simulink model "sim_all_2019b"  (R2019b)
settings: Solver=VariableStepAuto  StartTime=0.0  StopTime=2000  RelTol=1e-3
values from neighbouring files (symbols this model uses):
  nav_DT = 0.1    [navigation.m]
  nav_giro = 2    [navigation.m]
  nav_h0 = 0    [navigation.m]
  nav_lat0 = cornerC(1)    [navigation.m]
  nav_lon0 = cornerC(2)    [navigation.m]
  nav_plane_AB = coefficient_plane(nav_A,nav_B)    [navigation.m]
  nav_plane_BC = coefficient_plane(nav_B,nav_C)    [navigation.m]
  nav_plane_CD = coefficient_plane(nav_C,nav_D)    [navigation.m]
  nav_plane_DA = coefficient_plane(nav_D,nav_A)    [navigation.m]
undefined symbols (not defined in the file or in its folder): a1, a2, alpha1, alpha2, cornerA, cornerB, cornerC, cornerD, ctrl_clockwise, ctrl_int_bound_or, ctrl_int_bound_pos, ctrl_k_or, ctrl_k_pos, ctrl_Ki_vel, ctrl_Kp_v_pos, ctrl_Kp_vel, ctrl_TAM, ctrl_Ts, ctrl_va_uncontrolled, ctrl_vel_uncontrolled, D, dead_zone_limit, depth, DiscIntNeverNeededParam, distanceFromWall, initInspectedSide, initPoint, mod_A, mod_Cd_F, mod_Cd_M, mod_eta_init, mod_g, mod_h0, mod_Ixx, mod_Iyy, mod_Izz, mod_Kp_dot, mod_lat0, mod_lon0, mod_m, mod_Mq_dot, mod_ni_init, mod_Nr_dot, mod_p1, mod_p2, mod_p3, mod_p4, mod_p5, mod_p6, mod_R, mod_Rm, mod_t1, mod_t2, mod_t3, mod_t4, mod_t5, mod_t6, mod_W, mod_Xu_dot, mod_Yv_dot ... (+44)
libraries: simulink x8, cstblocks x6, simulink_extras x1
(part 4 of 6)

== matlab function sim_all_2019b/Mission_supervisor_v3/Mission_Supervisor/Completamento/MATLAB Function ==
  data: delta_current_comp output; parete input; delta_stato_comp output; Pos_d output size=3; Vel_d output; Dpp_d output; Orp_d output; Pos_s input; Vel_s input; Dpp_s input; Dps_s input; Orp_s input; depth parameter; speed parameter; distanceFromWall parameter; relativeDirection parameter; dps_fin input; error_flag input; soglia_SOS_vel parameter; soglia_parete_frenata parameter; soglia_SOS_orp parameter; soglia_SOS_pos parameter; soglia_SOS_parete parameter; SOS parameter; giro input
function [delta_current_comp, delta_stato_comp, Pos_d, Vel_d, Dpp_d, Orp_d] = Completamento(parete, Pos_s, Vel_s, Dpp_s, Dps_s, Orp_s, depth, speed, distanceFromWall, relativeDirection, dps_fin, error_flag, soglia_SOS_vel, soglia_parete_frenata, soglia_SOS_orp, soglia_SOS_pos, soglia_SOS_parete, SOS, giro)

    disp("Completamento del pattugliamento parziale della parete " + parete);
    
    %% Unità di misura 
    
    % Pos_d, Pos_s, soglia_SOS_pos                                                                              [deg, deg, m]
    % Orp_d, Orp_s, soglia_SOS_orp                                                                              [rad]
    % relativeDirection                                                                                         [deg]
    % Dpp_d, Dps_d, Dpp_s, Dps_s, dps_fin, distanceFromWall, depth, soglia_SOS_parete, soglia_parete_frenata    [m]
    % Vel_d, Vel_s, speed, soglia_SOS_vel                                                                       [m/s]

    %% Inizializzazione variabili
    
    % Utilizzata per permanere in questo stato e inizializzata a zero
    % perché fuori dal ciclo
    delta_stato_comp = 0; 
    
    pronti = false;
    
    
    %% Preparazione dei riferimenti da fornire ai blocchi successivi
    
    % Profondità da mantenere
    Pos_d = [nan; nan; depth];
                                                                            %*****TEST******%
                                                                            %Pos_d = [nan; nan; 0];
    
    % Velocità da raggiungere
    Vel_d = speed;              
                                                                            %*****TEST******%
                                                                            %Vel_d_vett = [0; 0; 0];

    % Distanza dalla parete da mantenere
    Dpp_d = distanceFromWall;
    
    % Orientazione da mantenere
    Orp_d = deg2rad(relativeDirection);
        
    % Transizione di stato effettiva
    delta_current_comp = 204 - 203;  
  
    %% Verifiche
    
    % Verifica sulla corretta profondità, orientazione, distanza dalla parete pattugliata 
    % e velocità
    if (abs(Pos_s(3) - Pos_d(3)) > soglia_SOS_pos(3) || ...
        abs(Orp_s - Orp_d) > soglia_SOS_orp || ...
        abs(Dpp_s - Dpp_d) > soglia_SOS_parete || ...
        norm(Vel_s) - Vel_d > soglia_SOS_vel)
    
        SOS = 1;
        disp("EMERGENZA:");
        
        if (abs(Orp_s - Orp_d) > soglia_SOS_orp)
            disp("Rilevato errore sull'orientazione relativa");
        end
        
        if (abs(Dpp_s - Dpp_d) > soglia_SOS_parete)
            disp("Rilevato errore sulla distanza da parete");
        end
        
        if (abs(Pos_s(3) - Pos_d(3)) > soglia_SOS_pos(3))
            disp("Rilevato errore sulla profondita Z");
        end
        
        if (norm(Vel_s) - Vel_d > soglia_SOS_vel)
            disp("Rilevato errore nella velocita");
        end

    end
    
                                                                            %*****TEST******%
                                                                            % if(contatore > 1)
                                                                            %     error_flag = 1;
                                                                            % end

     if error_flag == 1
        disp("EMERGENZA: errore segnalato dagli altri sottosistemi");
        SOS = 1;
     end
     
                                                                            %*****TEST******%
                                                                            %dps_fin = 4;

    % Si verifica di pattugliare alla velocità desiderata fino al punto di
    % frenata
    if (SOS == 0 && ...
        abs(Dps_s - (dps_fin + 3*speed)) < soglia_parete_frenata) % Analogo a quanto detto in "Pattugliamento"
    
        pronti = true;
        
    end
    
    %% Decisione dello stato successivo
    
    if pronti == true
        
        delta_stato_comp = 205 - 204; % Transizione eseguita correttamente
    end
    if SOS == 1
            
            delta_stato_comp = 301 - 204; % Transizione nello stato di emergenza
    end
  % Si rimane nello stato corrente.

end

== matlab function sim_all_2019b/Mission_supervisor_v3/Mission_Supervisor/Frenata in completamento/MATLAB Function ==
  data: delta_current_fren_comp output; delta_stato_fren_comp output; SOS_205 output; Pos_d output size=3; Dpp_d output; Dps_d output; Orp_d output; Pos_s input; Orp_s input; Dpp_s input; Dps_s input; depth parameter; distanceFromWall parameter; relativeDirection parameter; dps_fin input; error_flag input; soglia_SOS_pos parameter; soglia_SOS_parete parameter; soglia_SOS_orp parameter; soglia_parete parameter; SOS parameter
function [delta_current_fren_comp, delta_stato_fren_comp, SOS_205, Pos_d, Dpp_d, Dps_d, Orp_d] = Frenata_completamento(Pos_s, Orp_s, Dpp_s, Dps_s, depth, distanceFromWall, relativeDirection, dps_fin, error_flag, soglia_SOS_pos, soglia_SOS_parete, soglia_SOS_orp, soglia_parete, SOS)

    disp("Frenata (durante il completamento del pattugliamento parziale)");
    
    %% Unità di misura 
    
    % Pos_d, Pos_s, soglia_SOS_pos                                                                      [deg, deg, m]
    % Orp_d, Orp_s, soglia_SOS_orp                                                                      [rad]
    % relativeDirection                                                                                 [deg]
    % Dpp_d, Dps_d, Dpp_s, Dps_s, dps_fin, distanceFromWall, depth, soglia_SOS_parete, soglia_parete    [m]
    
    %% Inizializzazione variabili
    
    delta_stato_fren_comp = 0;
    
    pronti = false;
    

    %% Preparazione dei riferimenti da fornire si blocchi successivi
    
    % Profondità da mantenere
    Pos_d = [nan; nan; depth];
                                                                            %*****TEST******%
                                                                            %Pos_d = [nan;nan;0];
    % Distanza dalla parete da mantenere
    Dpp_d = distanceFromWall;
    Dps_d = dps_fin;
    
    % Orientazione da mantenere
    Orp_d = deg2rad(relativeDirection);
    
    % Transizione di stato effettiva
    delta_current_fren_comp = 205 - 204;  
    
       
    %% Verifiche

    % Si verifica la corretta orientazione, profondità e distanza dalla parete di pattugliamento 
    if (abs(Pos_s(3) - Pos_d(3)) > soglia_SOS_pos(3) || ...
        abs(Orp_s - Orp_d) > soglia_SOS_orp || ...
        abs(Dpp_s - Dpp_d) > soglia_SOS_parete)
    
        SOS = 1;
        pronti = true;
        disp("EMERGENZA:");
        
        if (abs(Pos_s(3) - Pos_d(3)) > soglia_SOS_pos(3))
            disp("Rilevato errore sulla profondita Z");
        end
        
        if (abs(Orp_s - Orp_d) > soglia_SOS_orp)
            disp("Rilevato errore sull'orientazione relativa");
        end
        
        if (abs(Dpp_s - Dpp_d) > soglia_SOS_parete)
            disp("Rilevato errore sulla distanza da parete");
        end
    end
    
    if error_flag == 1
        disp("EMERGENZA: errore segnalato dagli altri sottosistemi");
        SOS = 1;
    end
 
    SOS_205 = SOS;                                                                     %*****TEST******%
                                                                            %dps_fin = 8;

    % Si verifica di aver raggiunto la posizione desiderata di fine pattugliamento
    if (SOS==0 && ...
        abs(Dps_s - dps_fin) < soglia_parete) 
        pronti = true;
        
    end
    
    %% Decisione dello stato successivo
    
    if (pronti == true || SOS == 1)
        
        delta_stato_fren_comp = 301 - 205; % Transizione di stato
    end
    % Si rimane nello stato corrente
    

end

== matlab function sim_all_2019b/Mission_supervisor_v3/Mission_Supervisor/Orientazione in superficie/MATLAB Function ==
  data: delta_current_or_sup output; delta_stato_or_sup output; Or_in input; error_flag input; punto_iniz_patt input; SOS parameter; Pos_d output size=3; Or_d output size=3; soglia_SOS_pos parameter; soglia_or parameter; Pos_s input; Or_s input; soglia_SOS_or parameter
function [delta_current_or_sup, delta_stato_or_sup, Pos_d, Or_d] = Orientazioneinsuperficie(Or_in, error_flag, punto_iniz_patt, SOS, soglia_SOS_pos, soglia_or, Pos_s, Or_s, soglia_SOS_or)

    disp("Orientazione in superficie");
    
    %% Unità di misura 
    
    % Pos_d, Pos_s, soglia_SOS_pos, punto_iniz_patt                             [deg,deg,m]
    % Or_d, Or_in, Or_s, soglia_SOS_or, soglia_or                               [deg,deg,deg]

    %% Inizializzazione variabili
    
    delta_stato_or_sup = 0;
    
    pronti = false; 

    %% Preparazione dei riferimenti da fornire ai blocchi successivi
  
    % Posizione da mantenere
    Pos_d = punto_iniz_patt; 
                                                                            %*****TEST******%
                                                                            %Pos_d = [43; 11; 0];  
    % Orientazione desiderata e necessaria per raggiungere
    % il punto di rientro
    Or_d = Or_in;
                                                                            %*****TEST******%
                                                                            %Or_d = [1; 1; 1];
  
    % Transizione di stato effettiva
    delta_current_or_sup = 302 - 301;
   
    
    %% Verifiche 
    
    % Verifica della posizione e dell'orientazione
   if (abs(Pos_s(1) - Pos_d(1)) > soglia_SOS_pos(1) || ...
       abs(Pos_s(2) - Pos_d(2)) > soglia_SOS_pos(2) || ...
       abs(Pos_s(3) - Pos_d(3)) > soglia_SOS_pos(3) || ...
       abs(Or_s(1) - Or_d(1)) > soglia_SOS_or(1) || ...
       abs(Or_s(2) - Or_d(2)) > soglia_SOS_or(2))
    
        SOS = 1;
        disp("EMERGENZA:");
        
        
        if (abs(Pos_s(1) - Pos_d(1)) > soglia_SOS_pos(1))
            disp("Rilevato errore sulla posizione X");
        end
        if (abs(Pos_s(2) - Pos_d(2)) > soglia_SOS_pos(2))
            disp("Rilevato errore sulla posizione Y");
        end
        if (abs(Pos_s(3) - Pos_d(3)) > soglia_SOS_pos(3))
            disp("Rilevato errore sulla profondita Z");
        end
        if (abs(Or_s(1) - Or_d(1)) > soglia_SOS_or(1))
            disp("Rilevato errore sulla rotazione di roll");
        end
        if (abs(Or_s(2) - Or_d(2)) > soglia_SOS_or(2))
            disp("Rilevato errore sulla rotazione di pitch");
        end

    end
    
    if error_flag == 1
        disp("EMERGENZA: errore segnalato dagli altri sottosistemi");
        SOS = 1;
    end
    
    % Si verifica di aver raggiunto l'orientazione desiderata
    if  (SOS == 0 && ...
         abs(Or_s(3) - Or_d(3)) < soglia_or(3))
    
        pronti = true;
        
    end
    
%% Decisione dello stato successivo
    
    if pronti == true
       
        delta_stato_or_sup = 303 - 302; % Transizione eseguita correttamente
    end
    
    if SOS == 1
            
            delta_stato_or_sup = 304 - 302; % Transizione nello stato di emergenza
    end

    % Si rimane nello stato corrente
end

== matlab function sim_all_2019b/Mission_supervisor_v3/Mission_Supervisor/Pattugliamento/MATLAB Function ==
  data: parete input; contatore input; delta_current_patt output; Pos_s input; Dpp_s input; Dps_s input; delta_stato_patt output; Pos_d output size=3; Vel_d output; Dpp_d output; Orp_d output; Orp_s input; Vel_s input; depth parameter; speed parameter; distanceFromWall parameter; relativeDirection parameter; soglia_parete_frenata parameter; soglia_SOS_orp parameter; soglia_SOS_parete parameter; soglia_SOS_pos parameter; error_flag input; SOS parameter; soglia_SOS_vel parameter; giro input
function [delta_current_patt, delta_stato_patt, Pos_d, Vel_d, Dpp_d, Orp_d] = Pattugliamento(parete, contatore, Pos_s, Dpp_s, Dps_s, Orp_s, Vel_s, depth, speed, distanceFromWall, relativeDirection, soglia_parete_frenata, soglia_SOS_orp, soglia_SOS_parete, soglia_SOS_pos, error_flag, SOS, soglia_SOS_vel, giro)
    
    % In base al valore del contatore un display mostra il tipo di pattugliamento (parziale o completo)
    if contatore == 0
        disp("Pattugliamento parziale parete " + parete);
    else
        disp("Pattugliamento parete " + parete);
    end 
    
    %% Unità di misura 
    
    % Pos_d, Pos_s, soglia_SOS_pos                                                        [deg, deg, m]
    % Orp_d, Orp_s, soglia_SOS_orp                                                        [rad]
    % relativeDirection                                                                   [deg]
    % Dpp_d,Dpp_s, depth, distanceFromWall, soglia_parete_frenata, soglia_SOS_parete      [m]
    % Vel_d, Vel_s, speed, soglia_SOS_vel                                                 [m/s]

    
    %% Inizializzazione variabili
    
    % Si attribuisce alla variabile delta_stato_patt il valore contatore per  
    % tenere traccia delle transizioni effettuate durante il ciclo di
    % pattugliamento. Questo deve essere fatto perché i valori delta_stato
    % rimangono attivi una volta inizializzati nel ciclo.
    delta_stato_patt = contatore;
    
    pronti = false;
    
    %% Preparazione dei riferimenti da fornire ai blocchi successivi
    
    % Profondità da mantenere
    Pos_d = [nan; nan; depth];
                                                                            %*****TEST******%
                                                                            %Pos_d = [nan;nan;0];
    
    % Velocità da raggiungere
    Vel_d = speed;             

    % Distanza dalla parete da mantenere
    Dpp_d = distanceFromWall;
    
    % Orientazione da mantenere
    Orp_d = deg2rad(relativeDirection);
    
    
    % Transizione di stato effettiva a seconda che si arrivi da
    % "Orientazione in profondità" o da "Manovra"
    delta_current_patt = 201-104;   
   
    if contatore>0
        delta_current_patt = 201 - 104 - (2*contatore); 
    end
       
    %% Verifiche
    
    %Verifica sull'orientazione, sulla velocità, sulla profondità e sulla
    %distanza dalla parete pattugliata
    if (abs(Pos_s(3) - Pos_d(3)) > soglia_SOS_pos(3) || ...
        abs(Orp_s - Orp_d) > soglia_SOS_orp || ...
        norm(Vel_s) - Vel_d > soglia_SOS_vel || ...
        abs(Dpp_s - Dpp_d) > soglia_SOS_parete)
 
        SOS = 1;
        disp("EMERGENZA:");
        
        if (abs(Orp_s-Orp_d) > soglia_SOS_orp)
            disp("Rilevato errore sull'orientazione relativa");
        end
        if (abs(Dpp_s - Dpp_d) > soglia_SOS_parete)
            disp("Rilevato errore sulla distanza da parete");
        end
        if (abs(Pos_s(3) - Pos_d(3)) > soglia_SOS_pos(3))
            disp("Rilevato errore sulla profondita");
        end
        if (norm(Vel_s) - Vel_d > soglia_SOS_vel)
            disp("Rilevato errore sulla velocita");
        end

    end
%                                                                             %*****TEST******%
%                                                                             if(contatore>1)
%                                                                                 error_flag=1;
%                                                                             end

     if error_flag == 1
        disp("EMERGENZA: errore segnalato dagli altri moduli");
        SOS = 1;
     end
                                                                            %*****TEST******%
                                                                            %Serve per testare di rimanere 
                                                                            %in attesa in questo stato 
                                                                            %test=0;
%                                                                             if(contatore>1)%test
%                                                                                test=100;
%                                                                             else
%                                                                                test=0;
%                                                                             end
    
    % Si verifica di pattugliare fino al punto di frenata calcolata
    % considerando un tempo di frenata di tre secondi
    if (SOS == 0 && ...
        abs(Dps_s - (distanceFromWall + 3*speed)) < soglia_parete_frenata) 

        
        pronti = true;
        
    end
    
    %% Decisione dello stato successivo
    
    if pronti == true

        delta_stato_patt = 202 - 201 + contatore; %Transizione eseguita correttamente
    end
    if SOS == 1
            
            delta_stato_patt = 301 - 201 + contatore; %Transizione nello stato di emergenza
    end
% Si rimane nello stato corrente

end

== matlab function sim_all_2019b/Mission_supervisor_v3/Mission_Supervisor/Fine missione/MATLAB Function ==
  data: delta_current_end output; stato input
function delta_current_end  = Fine_missione(stato)

    disp("Fine missione");
    
    
    
    %% Transizione di stato effettiva 
    delta_current_end = 304 - stato;  
    
    % La missione è conclusa e la simulazione termina.

end

== matlab function sim_all_2019b/Mission_supervisor_v3/Mission_Supervisor/Posizionamento/MATLAB Function ==
  data: delta_current_posiz output; delta_stato_posiz output; Pos_d output size=3; Or_d output size=3; Pos_s input; Or_s input; punto_iniziale input; Or_in input; error_flag input; soglia_pos parameter; soglia_SOS_or parameter; SOS parameter; soglia_SOS_pos parameter
function [delta_current_posiz, delta_stato_posiz, Pos_d, Or_d] = Posizionamento(Pos_s, Or_s, punto_iniziale, Or_in, error_flag, soglia_pos, soglia_SOS_or, SOS, soglia_SOS_pos)

    disp("Posizionamento");
    
    %% Unità di misura 
    
    % Pos_d, Pos_s, punto_iniziale, soglia_pos, soglia_SOS_pos             [deg, deg, m]
    % Or_d, Or_s, Or_in, soglia_SOS_or                                     [rad, rad, rad]

    %% Inizializzazione variabili
    
    % Mantenimento dello stato_interno al valore
    % desiderato durante la permanenza del sistema nello stato corrente.
    delta_stato_posiz = 0;
    
    pronti = false;
   
    %% Preparazione dei riferimenti da fornire ai blocchi successivi
    
    % Posizione da raggiungere
    Pos_d = punto_iniziale;                                                %*****TEST******%
                                                                            %Pos_d = [43; 11; 0];
     
   
    % Orientazione da mantenere
    Or_d = Or_in;
    
    % Transizione di stato effettiva
    delta_current_posiz = 102 - 101;  
       
    
    %% Verifiche
    
     % Verifica della corretta orientazione e profondità
     
    if (abs(Or_s(1) - Or_d(1)) > soglia_SOS_or(1) || ...
        abs(Or_s(2) - Or_d(2)) > soglia_SOS_or(2) || ...
        abs(Or_s(3) - Or_d(3)) > soglia_SOS_or(3) || ...
        abs(Pos_s(3) - Pos_d(3)) > soglia_SOS_pos(3))
    
        SOS = 1;
        disp("EMERGENZA:");       
        
        if (abs(Or_s(1) - Or_d(1)) > soglia_SOS_or(1))
            disp("Rilevato errore sulla rotazione di roll");
        end
        
        if (abs(Or_s(2) - Or_d(2)) > soglia_SOS_or(2))
            disp("Rilevato errore sulla rotazione di pitch");
        end
        
        if (abs(Or_s(3) - Or_d(3)) > soglia_SOS_or(3))
            disp("Rilevato errore sulla rotazione di yaw");
        end
       
        if (abs(Pos_s(3) - Pos_d(3)) > soglia_SOS_pos(3))
            disp("Rilevato errore sulla posizione lungo z");
        end
        
    end
    
    if error_flag == 1
        disp("EMERGENZA: errore segnalato dagli altri sottosistemi");
        SOS = 1;
    end
    
    % Si verifica di aver raggiunto la posizione desiderata
    if (SOS == 0 && ...
        abs(Pos_s(1) - Pos_d(1)) < soglia_pos(1) && ...
        abs(Pos_s(2) - Pos_d(2)) < soglia_pos(2))
    
        pronti = true;
        
    end

    %% Decisione dello stato successivo
     
    if pronti == true
        
        delta_stato_posiz = 103 - 102; % Transizione eseguita correttamente
    end
    if SOS == 1
            
            delta_stato_posiz = 304 - 102; % Transizione nello stato di emergenza
    end
    % Si rimane nello stato corrente

end

== matlab function sim_all_2019b/Mission_supervisor_v3/Mission_Supervisor/Rientro/MATLAB Function ==
  data: delta_current_rient output; delta_stato_rient output; Pos_d output size=3; Pos_s input; initPoint parameter; Or_in input; Or_d output size=3; soglia_pos parameter; SOS parameter; error_flag input; Dps_s input; Dpp_s input; soglia_SOS_collisione parameter; soglia_SOS_or parameter; soglia_SOS_pos parameter; Or_s input
function [delta_current_rient, delta_stato_rient, Pos_d, Or_d] = Rientro(Pos_s, initPoint, Or_in, soglia_pos, SOS, error_flag, Dps_s, Dpp_s, soglia_SOS_collisione, soglia_SOS_or, soglia_SOS_pos, Or_s)

    disp("Rientro");
    
    %% Unità di misura 
    
    % Pos_d, Pos_s, soglia_pos, initPoint, soglia_SOS_pos                    [deg,deg,m]
    % Or_d, Or_in, Or_s, soglia_SOS_or                                       [deg,deg,deg]
    % Dps_s, Dpp_s, soglia_SOS_collisione_s                                  [m]

    %% Inizializzazione variabili
    
    delta_stato_rient = 0;
    
    pronti = false;
    
    %% Preparazione dei riferimenti da fornire ai blocchi successivi
      
    % Posizione da raggiungere
    Pos_d = initPoint;
    
    % Orientazione da mantenere
    Or_d = Or_in;
    
    % Transizione di stato effettiva
    delta_current_rient = 303 - 302; 
       
    %% Verifiche
    
    % Verifica sulla profondità, sull'orientazione e sull'assenza di collisioni
    if (Dpp_s  < soglia_SOS_collisione || ... 
        Dps_s < soglia_SOS_collisione || ...
        abs(Or_s(1) - Or_d(1)) > soglia_SOS_or(1) || ...
        abs(Or_s(2) - Or_d(2)) > soglia_SOS_or(2) || ...
        abs(Or_s(3) - Or_d(3)) > soglia_SOS_or(3) || ...
        abs(Pos_s(3) - Pos_d(3)) > soglia_SOS_pos(3))
            
    
        SOS = 1;
        disp("EMERGENZA:");  
 

        if (Dpp_s < soglia_SOS_collisione || ... 
            Dps_s < soglia_SOS_collisione)
            disp("Pericolo collisione");
        end
        
        if (abs(Or_s(1) - Or_d(1)) > soglia_SOS_or(1))
            disp("Rilevato errore sulla rotazione di roll");
        end
        
        if (abs(Or_s(2) - Or_d(2)) > soglia_SOS_or(2))
            disp("Rilevato errore sulla rotazione di pitch");
        end
        
        if (abs(Or_s(3) - Or_d(3)) > soglia_SOS_or(3))
            disp("Rilevato errore sulla rotazione di yaw");
        end
     
        if (abs(Pos_s(3) - Pos_d(3)) > soglia_SOS_pos(3))
            disp("Rilevato errore sulla posizione lungo z");
        end
    
    end
    
    if error_flag == 1
        
        disp("EMERGENZA: errore segnalato dagli altri sottosistemi");
        SOS = 1;
        
    end
   
    % Si verifica di aver raggiunto la posizione desiderata
    if (SOS == 0 && ...
        abs(Pos_s(1) - Pos_d(1)) < soglia_pos(1) && ...
        abs(Pos_s(2) - Pos_d(2)) < soglia_pos(2))
    
        pronti = true;
        
    end
    

    
   %% Decisione dello stato successivo
    
   % Si effettua la transizione nello stato successivo indipendentemente
   % dal verificarsi di una emergenza
    if (pronti == true || SOS == 1)

        delta_stato_rient = 304 - 303;
    end
    % Si rimane nello stato corrente

end

== matlab function sim_all_2019b/Controller_mk4_v3/C_or/C_or_X ==
  data: err_int output; ang input; vel output; k input; ctrl_va_uncontrolled parameter; ctrl_int_bound_or parameter
%% Azione proporzionale
function [err_int, vel] = fcn(ang, k, ctrl_va_uncontrolled, ctrl_int_bound_or)
    v = 0;
    err_int = 0;
    va_des = ctrl_va_uncontrolled;  % velocità impostata prima della fase di frenata
    brake_dist = (1/k)*va_des;      % distanza in cui dobbiamo iniziare a frenare
    if ang >= brake_dist            % al di fuori dello spazio di frenata
        v = va_des;
    end
    if ang <= -brake_dist           % al di fuori dello spazio di frenata in negativo
        v = -va_des;
    end
    if  abs(ang) < brake_dist       % proporzionale se entro la distanza di frenata
        v = k*ang;
    end
    vel = v;
    if abs(ang) < ctrl_int_bound_or    % per il regime può essere utile una azione integrale
        err_int = ang;                 % err_int va ad un integratore
    end
end

== matlab function sim_all_2019b/Controller_mk4_v3/C_or/C_or_Y ==
  data: err_int output; ang input; vel output; k input; ctrl_va_uncontrolled parameter; ctrl_int_bound_or parameter
%% Azione proporzionale
function [err_int, vel] = fcn(ang, k, ctrl_va_uncontrolled, ctrl_int_bound_or)
    v = 0;
    err_int = 0;
    va_des = ctrl_va_uncontrolled;  % velocità impostata prima della fase di frenata
    brake_dist = (1/k)*va_des;      % distanza in cui dobbiamo iniziare a frenare
    if ang >= brake_dist            % al di fuori dello spazio di frenata
        v = va_des;
    end
    if ang <= -brake_dist           % al di fuori dello spazio di frenata in negativo
        v = -va_des;
    end
    if  abs(ang) < brake_dist       % proporzionale se entro la distanza di frenata
        v = k*ang;
    end
    vel = v;
    if abs(ang) < ctrl_int_bound_or    % per il regime può essere utile una azione integrale
        err_int = ang;                 % err_int va ad un integratore
    end
end

== matlab function sim_all_2019b/Controller_mk4_v3/C_or/C_or_Z ==
  data: err_int output; ang input; vel output; k input; ctrl_va_uncontrolled parameter; ctrl_int_bound_or parameter
%% Azione proporzionale
function [err_int, vel] = fcn(ang, k, ctrl_va_uncontrolled, ctrl_int_bound_or)
    v = 0;
    err_int = 0;
    va_des = ctrl_va_uncontrolled;  % velocità impostata prima della fase di frenata
    brake_dist = (1/k)*va_des;      % distanza in cui dobbiamo iniziare a frenare
    if ang >= brake_dist            % al di fuori dello spazio di frenata
        v = va_des;
    end
    if ang <= -brake_dist           % al di fuori dello spazio di frenata in negativo
        v = -va_des;
    end
    if  abs(ang) < brake_dist       % proporzionale se entro la distanza di frenata
        v = k*ang;
    end
    vel = v;
    if abs(ang) < ctrl_int_bound_or    % per il regime può essere utile una azione integrale
        err_int = ang;                 % err_int va ad un integratore
    end
end

== matlab function sim_all_2019b/Controller_mk4_v3/C_pos/C_pos_X ==
  data: err_int output; pos input; vel output; k input; ctrl_vel_uncontrolled parameter; ctrl_int_bound_pos parameter
%% Azione proporzionale
function [err_int, vel] = fcn(pos, k, ctrl_vel_uncontrolled, ctrl_int_bound_pos)
    v = 0;
    err_int = 0;
    vel_des = ctrl_vel_uncontrolled;    % velocità impostata se 'lontani'
    brake_dist = 1/k*vel_des;           % distanza di frenata
    if pos >= brake_dist                % se ho spazio per frenare mantengo la velocità
        v = vel_des;
    end
    if pos <= -brake_dist               % lontani in direzione negativa
        v = -vel_des;
    end
    if  abs(pos) < brake_dist           % se è vicino il proporzionale gestisce la frenata
        v = k*pos;
    end
    vel = v;
    if abs(pos) < ctrl_int_bound_pos    % per il regime può essere utile una azione integrale
        err_int = pos;                  % err_int va ad un integratore
    end

== matlab function sim_all_2019b/Controller_mk4_v3/C_pos/C_pos_Z ==
  data: err_int output; pos input; vel output; k input; ctrl_vel_uncontrolled parameter; ctrl_int_bound_pos parameter
%% Azione proporzionale
function [err_int, vel] = fcn(pos, k, ctrl_vel_uncontrolled, ctrl_int_bound_pos)
    v = 0;
    err_int = 0;
    vel_des = ctrl_vel_uncontrolled;    % velocità impostata se 'lontani'
    brake_dist = 1/k*vel_des;           % distanza di frenata
    if pos >= brake_dist                % se ho spazio per frenare mantengo la velocità
        v = vel_des;
    end
    if pos <= -brake_dist               % lontani in direzione negativa
        v = -vel_des;
    end
    if  abs(pos) < brake_dist           % se è vicino il proporzionale gestisce la frenata
        v = k*pos;
    end
    vel = v;
    if abs(pos) < ctrl_int_bound_pos    % per il regime può essere utile una azione integrale
        err_int = pos;                  % err_int va ad un integratore
    end

== matlab function sim_all_2019b/Controller_mk4_v3/InputOr_Organizer/diff_or ==
  data: or_d input; err_or output; or_s input
%% Calcolo errore
function err_or = fcn(or_d, or_s)
coder.extrinsic('wrapToPi');
err_or = zeros(3,1);
err_or = wrapToPi(or_d - or_s);    % rimane compreso tra -pi e +pi
end

== matlab function sim_all_2019b/Controller_mk4_v3/InputPos_Organizer/Ned2Body1 ==
  data: x_n input size=[3 1]; x_b output size=[3 1]; or input
%% Da NED a BODY
function x_b = ned2body(x_n,or)
C=zeros(3,3);
C=Cx(or(1))'*Cy(or(2))'*Cz(or(3))';
x_b = C'*x_n;
end

== matlab function sim_all_2019b/Controller_mk4_v3/InputPos_Organizer/Ned2Body2 ==
  data: x_n input size=[3 1]; x_b output size=[3 1]; or input
%% Da NED a BODY
function x_b = ned2body(x_n,or)
C=zeros(3,3);
C=Cx(or(1))'*Cy(or(2))'*Cz(or(3))';
x_b = C'*x_n;
end

== matlab function sim_all_2019b/Navigation/Extended Kalman Filter/MATLAB Function5 ==
  data: u input; dev_standard_x output; dev_standard_y output; dev_standard_z output
function [dev_standard_x,dev_standard_y,dev_standard_z] = fcn(u) 
    
    dev_standard_x = sqrt(u(1,1));
    dev_standard_y = sqrt(u(2,2));
    dev_standard_z = sqrt(u(3,3));
end

== matlab function sim_all_2019b/Controller_mk4_v3/InputPos_Organizer/Ned2Body3 ==
  data: x_n input size=[3 1]; x_b output size=[3 1]; or input
%% Da NED a BODY
function x_b = ned2body(x_n,or)
C=zeros(3,3);
C=Cx(or(1))'*Cy(or(2))'*Cz(or(3))';
x_b = C'*x_n;
end

== matlab function sim_all_2019b/Controller_mk4_v3/InputPos_Organizer/Ned2Body4 ==
  data: x_n input size=[3 1]; x_b output size=[3 1]; or input
%% Da NED a BODY
function x_b = ned2body(x_n,or)
C=zeros(3,3);
C=Cx(or(1))'*Cy(or(2))'*Cz(or(3))';
x_b = C'*x_n;
end

== matlab function sim_all_2019b/Controller_mk4_v3/InputPos_Organizer/brake_trigger ==
  data: state input; trigg_brake output
%% Restituisce 0 se in frenata
% In frenata vengono controllate sia dpp che dps
function trigg_brake = fcn(state)
tmp = 0;
switch state
    case 100            % fermo in superficie
        tmp = 1;
    case 101            % orientazione verso parete di inizio in superficie
        tmp = 1;
    case 102            % posizionamento in superficie
        tmp = 1;   
    case 103            % immersione
        tmp = 1;
    case 104            % orientazione in profondità
        tmp = 1;
    case 201            % pattugliamento
        tmp = 1;
    case 202            % frenata
        tmp = 0;
    case 203            % manovra di cambio parete
        tmp = 0;
    case 204            % competamento del pattugliamento della parete iniziale
        tmp = 1;
    case 205            % frenata a metà parete
        tmp = 0;
    case 301            % risalita
        tmp = 0;
    case 302            % orientazione in superficie
        tmp = 1;
    case 303            % rientro, ritorno al punto iniziale in superficie
        tmp = 1;
    case 304            % fine missione, tutto spento
        tmp = 1;
end
trigg_brake = tmp;
end

== matlab function sim_all_2019b/Controller_mk4_v3/InputVel_Organizer/Ned2Body4 ==
  data: x_n input size=[3 1]; x_b output size=[3 1]; or input
%% Da NED a BODY
function x_b = ned2body(x_n,or)
C=zeros(3,3);
C=Cx(or(1))'*Cy(or(2))'*Cz(or(3))';
x_b = C'*x_n;
end

== matlab function sim_all_2019b/Controller_mk4_v3/Mixer/Mix ==
  data: Tp input; T output; Tv input; To input; ctrl_T_max parameter
%% funzione che permette di gestire le saturazioni dei motori
function T = Mix(Tp, Tv, To, ctrl_T_max)
    T_sat = [   ctrl_T_max   ctrl_T_max   ctrl_T_max   ctrl_T_max   ctrl_T_max   ctrl_T_max;...
               -ctrl_T_max  -ctrl_T_max  -ctrl_T_max  -ctrl_T_max  -ctrl_T_max  -ctrl_T_max];
    tmp = Tp + Tv + To;
    freg = sumSat(ctrl_T_max, tmp);                 % freg indica se il vettore è da regolare
    if freg == true
        if sumSat(ctrl_T_max, To+Tp) == false       % caso in cui To+Tp non satura
            T_tmp = To + Tp;
            [T_sat, T_new] = prior(T_sat, T_tmp);
            [T_sat, T_new] = prior(T_sat, Tv);
            T = T_tmp + T_new;
        else                                        % caso generale, ridimensiona tutti i vettori che fanno saturare
            T_tmp = 0;
            [T_sat, T_new] = prior(T_sat, To);
            T_tmp = T_tmp + T_new;
            [T_sat, T_new] = prior(T_sat, Tp);
            T_tmp = T_tmp + T_new;
            [T_sat, T_new] = prior(T_sat, Tv);
            T = T_tmp + T_new;
        end
    else
        T = tmp;
    end
end

% sumSat() restituisce 1 se il vettore T_in supera la saturazione, è solo
% un controllo iniziale in quanto controlla solo se la somma delle spinte
% rientra in T_max
function resp = sumSat(T_max, T_in)
    tmp = false;
    for i=1:length(T_in)
        if abs(T_in(i)) > T_max
            tmp = true;
        end
    end
    resp = tmp;
end

% prior() prende vettore in ingresso e vettore delle saturazioni e
% restituisce vettore in ingresso ridimensionato e nuovo vettore delle
% saturazioni
function [T_sat_new, T_reg] = prior(T_sat, T_new)
    T_sat_tmp = T_sat;
    recalc = false;                 % serve per sapere se bisogna ricalcolare le precedenti saturazioni
    for i = 1:length(T_new)         % ciclo per calcolare i nuovi vettori ridimensionati
        if T_new(i)>0               % azione del motore positiva
            tmp = T_sat_tmp(1,i) - T_new(i);        % nuova saturazione temporanea
            if tmp < 0
                if i < 5                            % devo scalare i primi 4 motori per mantenere la direzione
                    k = abs(T_sat_tmp(1,i)/T_new(i));
                    T_new(1:4) = T_new(1:4) * k;
                    if i~=1                 % devo riaggiustare le T_sat precedenti se il motore che satura non è il primo
                        recalc = true;      % riaggiusto i T_sat in prior2
                    end
                else
                    k = abs(T_sat_tmp(1,i)/T_new(i));
                    j = ((floor(i/2.1)+1)*2);           % escamotage per prendere le coppie giuste, era per le coppie
                    T_new(j-1:j) = T_new(j-1:j) * k;    % ridimensiono le componenti relative al grado di libertà
                    if mod(i, 2) == 0                   % devo riaggiustare la T_sat precedente se i pari
                        recalc = true;                  % riaggiusto gli T_sat
                    end
                end
            end
            T_sat_tmp(1,i) = T_sat_tmp(1,i) - T_new(i);
            T_sat_tmp(2,i) = T_sat_tmp(2,i) - T_new(i);
        elseif T_new(i)<0                           % è identico al codice per T>0 ma speculare
            tmp = T_sat_tmp(2,i) - T_new(i);
            if tmp > 0
                if i < 5                            % devo scalare i primi 4 motori
                    k = abs(T_sat_tmp(2,i)/T_new(i));
                    T_new(1:4) = T_new(1:4) * k;
                    if i~=1                         % devo riaggiustare le T_sat precedenti se i 
                        recalc = true;              % riaggiusto gli T_sat
                    end
                else
                    k = abs(T_sat_tmp(2,i)/T_new(i));
                    j = (floor(i/2.1)+1)*2;     % escamotage per prendere le coppie giuste
                    T_new(j-1:j) = T_new(j-1:j) * k;
                    if mod(i, 2) == 0           % devo riaggiustare la T_sat precedente se i pari
                        recalc = true;          % riaggiusto gli T_sat
                    end
                end
            end
            T_sat_tmp(2,i) = T_sat_tmp(2,i) - T_new(i);
            T_sat_tmp(1,i) = T_sat_tmp(1,i) - T_new(i);
        end
    end
    if recalc == true
        % devo rifare il ciclo con i nuovi T_new
        [T_sat_tmp, T_new] = prior2(T_sat, T_new);
    end
    T_sat_new = T_sat_tmp;      % T_sat_new è il nuovo vettore delle saturazioni
    T_reg = T_new;              % T_reg è il nuovo vettore scalato
end

% prior2() aggiusta il vettore delle saturazioni T_sat, uso interno a
% prior()
function [T_sat_new, T_reg] = prior2(T_sat, T_new)
    T_sat_tmp = T_sat;
    for i = 1:length(T_new)        % ciclo per calcolare quanti giri rimanenti prima di saturare
        if T_new(i)>0              % azione del motore positiva
            tmp = T_sat_tmp(1,i) - T_new(i);       % nuova saturazione temporanea
            T_sat_tmp(1,i) = tmp;
            T_sat_tmp(2,i) = T_sat_tmp(2,i) - T_new(i);
        else
            tmp = T_sat_tmp(2,i) - T_new(i);
            T_sat_tmp(2,i) = tmp;
            T_sat_tmp(1,i) = T_sat_tmp(1,i) - T_new(i);
        end
    end
    T_sat_new = T_sat_tmp;
    T_reg = T_new;
end

== matlab function sim_all_2019b/Controller_mk4_v3/Mixer/T2n ==
  data: T input size=[6 1]; n output; a1 parameter
%% Conversione da T a n
% Si usa relazione inclusa nel modello dei propulsiori
% sfruttando approssimazione quadratica
function n = T2n(T,a1)
n = zeros(6,1);
    for i= 1:length(T)
        if T(i) > 0
            n(i) = sqrt(T(i)/a1);
        else
            n(i) = -sqrt(-T(i)/a1);
        end
    end
end

== matlab function sim_all_2019b/Controller_mk4_v3/enabler ==
  settings: updateMethod=DISCRETE  sampleTime=ctrl_Ts
  data: state input; en_pos output; en_vel output; en_or output
function [en_pos, en_vel, en_or] = fcn(state)
    en = [0 0 0];
    persistent state_prec        % reset dell'azione integrale
    if isempty(state_prec)
        state_prec = 0;
    end
    if state ~= state_prec
        en = [0 0 0];
        state_prec = state;
    else
        switch state
            case 100            % fermo in superficie
                en = [1 0 0];
            case 101            % orientazione verso parete di inizio in superficie
                en = [1 0 1];
            case 102            % posizionamento in superficie
                en = [1 0 1];   
            case 103            % immersione
                en = [1 0 1];
            case 104            % orientazione in profondità
                en = [1 0 1];
            case 201            % pattugliamento
                en = [1 1 1];
            case 202            % frenata, da verificare con gli altri
                en = [1 0 1];
            case 203            % manovra di cambio parete
                en = [1 0 1];
            case 204            % competamento del pattugliamento della parete iniziale
                en = [1 1 1];
            case 205            % frenata a metà parete
                en = [1 0 1];
            case 301            % risalita
                en = [1 0 1];
            case 302            % orientazione in superficie
                en = [1 0 1];
            case 303            % rientro, ritorno al punto iniziale in superficie
                en = [1 0 1];
            case 304            % fine missione, tutto spento
                en = [0 0 0];
        end
    end
    en_pos = en(1);
    en_vel = en(2);
    en_or = en(3);
end

== matlab function sim_all_2019b/Controller_mk4_v3/lld2Ned ==
  data: x_ecef input size=[3 1]; x_n output; cornerC parameter
%% Da LLD (riferimento posizione assoluta) a NED
function x_n = ToNed_Pos(x_ecef,cornerC)
x_n=zeros(3,1);
coder.extrinsic('evalin', 'wgs84Ellipsoid', 'geodetic2ned');
[pNorth,pEast,pDown] = geodetic2ned(x_ecef(1),x_ecef(2),x_ecef(3),cornerC(1),cornerC(2),0,wgs84Ellipsoid);
x_n=[pNorth;pEast;x_ecef(3)];

end

== matlab function sim_all_2019b/Model/Vehicle Model/Acceleration Computation ==
  data: inertialTerm input; ni_dot output; mod_m parameter; mod_Ixx parameter; mod_Iyy parameter; mod_Izz parameter; mod_Xu_dot parameter; mod_Yv_dot parameter; mod_Zw_dot parameter; mod_Kp_dot parameter; mod_Mq_dot parameter; mod_Nr_dot parameter
function ni_dot = fcn(inertialTerm, mod_m, mod_Ixx, mod_Iyy, mod_Izz, mod_Xu_dot, mod_Yv_dot, mod_Zw_dot, mod_Kp_dot, mod_Mq_dot, mod_Nr_dot)

% Si definisce la matrice di inerzia del corpo rigido:
Mrb = [ mod_m   0   0   0   0   0;
        0   mod_m   0   0   0   0;
        0   0   mod_m   0   0   0;
        0   0   0  mod_Ixx  0   0;
        0   0   0   0  mod_Iyy  0;
        0   0   0   0   0  mod_Izz ];

% Si definisce la matrice di inerzia dovuta ai termini di massa e inerzia
% aggiunti:
Ma = [ -mod_Xu_dot     0        0        0        0        0;
          0     -mod_Yv_dot     0        0        0        0;
          0        0     -mod_Zw_dot     0        0        0;
          0        0        0     -mod_Kp_dot     0        0;
          0        0        0        0     -mod_Mq_dot     0;
          0        0        0        0        0     -mod_Nr_dot ];

M = Mrb + Ma;

ni_dot = M\inertialTerm;

== matlab function sim_all_2019b/Model/Vehicle Model/Coriolis term ==
  data: ni_rel input; mod_m parameter; mod_Ixx parameter; mod_Iyy parameter; mod_Izz parameter; mod_Xu_dot parameter; mod_Yv_dot parameter; mod_Zw_dot parameter; mod_Kp_dot parameter; Cterm output; mod_Mq_dot parameter; mod_Nr_dot parameter
function Cterm  = fcn(ni_rel, mod_m, mod_Ixx, mod_Iyy, mod_Izz, mod_Xu_dot, mod_Yv_dot, mod_Zw_dot, mod_Kp_dot, mod_Mq_dot, mod_Nr_dot)

u_rel = ni_rel(1);
v_rel = ni_rel(2);
w_rel = ni_rel(3);
p_rel = ni_rel(4);
q_rel = ni_rel(5);
r_rel = ni_rel(6);

% Si definisce la matrice di Coriolis del corpo rigido:
Crb = [    0          0          0           0          mod_m*w_rel     -mod_m*v_rel;
           0          0          0       -mod_m*w_rel          0         mod_m*u_rel;
           0          0          0        mod_m*v_rel      -mod_m*u_rel         0;
           0       mod_m*w_rel   -mod_m*v_rel        0        mod_Izz*r_rel   -mod_Iyy*q_rel;
       -mod_m*w_rel       0       mod_m*u_rel   -mod_Izz*r_rel         0       mod_Ixx*p_rel;
        mod_m*v_rel   -mod_m*u_rel       0       mod_Iyy*q_rel   -mod_Ixx*p_rel         0    ];

% Si definiscono i termini di Coriolis dovuti alle masse a alle inerzie
% aggiunte:
Ca = [      0              0              0              0        -mod_Zw_dot*w_rel   mod_Yv_dot*v_rel;
            0              0              0         mod_Zw_dot*w_rel        0        -mod_Xu_dot*u_rel;
            0              0              0        -mod_Yv_dot*v_rel   mod_Xu_dot*u_rel        0;
            0        -mod_Zw_dot*w_rel   mod_Yv_dot*v_rel        0        -mod_Nr_dot*r_rel   mod_Mq_dot*q_rel;
       mod_Zw_dot*w_rel        0        -mod_Xu_dot*u_rel   mod_Nr_dot*r_rel        0        -mod_Kp_dot*p_rel;
      -mod_Yv_dot*v_rel   mod_Xu_dot*u_rel        0        -mod_Mq_dot*q_rel   mod_Kp_dot*p_rel        0       ];

C = Crb + Ca;

Cterm = C*ni_rel;

== matlab function sim_all_2019b/Model/Vehicle Model/Damping term ==
  data: ni_rel input; Dterm output; rho parameter; mod_Rm parameter; mod_A parameter; mod_Cd_F parameter; mod_Cd_M parameter
function Dterm = fcn(ni_rel, rho, mod_Rm, mod_A, mod_Cd_F, mod_Cd_M)

u_rel = ni_rel(1);
v_rel = ni_rel(2);
w_rel = ni_rel(3);
p_rel = ni_rel(4);
q_rel = ni_rel(5);
r_rel = ni_rel(6);

%Termine costante di Damping rispettivamente riferito alle forze e ai momenti
Dconst_F = 0.5*rho*mod_Cd_F*mod_A;
Dconst_M = 0.5*rho*mod_Cd_M*mod_A*mod_Rm*mod_Rm*mod_Rm;

% Si definiscono i termini diagonali della matrice di Damping:
D1 = Dconst_F*abs(u_rel)*u_rel;
D2 = Dconst_F*abs(v_rel)*v_rel;
D3 = Dconst_F*abs(w_rel)*w_rel;
D4 = Dconst_M*abs(p_rel)*p_rel;
D5 = Dconst_M*abs(q_rel)*q_rel; 
D6 = Dconst_M*abs(r_rel)*r_rel; 

Dterm = [D1; D2; D3; D4; D5; D6];

== matlab function sim_all_2019b/Model/Vehicle Model/Gravitational terms ==
  data: eta input; Gterm output; mod_W parameter; mod_z_cm parameter; mod_R parameter; rho parameter; mod_g parameter
function Gterm = fcn (eta, mod_W, mod_z_cm, mod_R, rho, mod_g)

% Si definisce il vettore delle forze e dei momenti gravitazionali 
% considerando una forza di galleggiamento variabile al variare del volume 
% del veicolo immerso.

z = eta(3);
phi = eta(4);
theta = eta(5);
 
% Si definisce la componente z del vettore posizione del centro di
% galleggiamento rispetto al centro di massa:
z_CB = -0.1;

% Caso di veicolo totalmente immerso:
if (z >= mod_R + mod_z_cm)
    G = [0; 0; 0; mod_z_cm*mod_W*cos(theta)*sin(phi); mod_z_cm*mod_W*sin(theta); 0];

% Caso di veicolo parzialmente immerso (forza di galleggiamento variabile):
elseif (z >= -(mod_R - mod_z_cm) && z < (mod_R + mod_z_cm))
    Vol_immerso = pi*((z+mod_R-mod_z_cm)^2)*(mod_R-((z+mod_R-mod_z_cm)/3));
    B = rho*mod_g*Vol_immerso;
    G = [(mod_W-B)*sin(theta); -(mod_W-B)*cos(theta)*sin(phi); -(mod_W-B)*cos(theta)*cos(phi); -z_CB*B*cos(theta)*sin(phi); -z_CB*B*sin(theta); 0];

% Caso di veicolo completamente emerso (condizione che non si deve verificare per nessun motivo):
else
    G = [mod_W*sin(theta); -mod_W*cos(theta)*sin(phi); -mod_W*cos(theta)*cos(phi); 0; 0; 0];    
end

Gterm = G;

== matlab function sim_all_2019b/Model/Vehicle Model/Kinematic Model ==
  data: eta input; ni input; eta_dot output
function eta_dot = fcn(eta, ni)

phi = eta(4);
theta = eta(5); 
psi = eta(6);

% Si definisce la matrice di rotazione J1 che mappa la velocità lineare in 
% terna body nella velocità lineare in terna NED: 
J1 = [ cos(psi)*cos(theta)   -sin(psi)*cos(phi) + (cos(psi)*sin(theta)*sin(phi))   (sin(psi)*sin(phi)) + (cos(psi)*cos(phi)*sin(theta));
       sin(psi)*cos(theta)   (cos(psi)*cos(phi)) + (sin(psi)*sin(theta)*sin(phi))  (-cos(psi)*sin(phi)) + (sin(psi)*sin(theta)*cos(phi));
      -sin(theta)             cos(theta)*sin(phi)                                   cos(theta)*cos(phi)                                  ];

% Si definisce la matrice J2 che mappa la velocità angolare in terna body
% nel vettore orientazione espresso in terna NED (J2 non è una matrice di 
% rotazione):
J2 = [ 1   sin(phi)*tan(theta)   cos(phi)*tan(theta);
       0   cos(phi)             -sin(phi);
       0   sin(phi)/cos(theta)   cos(phi)/cos(theta) ];
       
J = [   J1      zeros(3);
      zeros(3)    J2     ];

eta_dot = J*ni;

== matlab function sim_all_2019b/Model/Vehicle Model/P1/Propeller1 ==
  data: n1 input; T1 output; V1 input; D parameter; omega parameter; a1 parameter; a2 parameter; alpha1 parameter; alpha2 parameter
function T1 = thrusterModel(n1, V1, D, omega, a1, a2, alpha1, alpha2)

Va1 = (1-omega) * V1;     % Advancement velocity at the propeller
J0 = Va1/(n1*D);          % Advancement Coefficient

if J0 > -alpha1/alpha2  % Out of linearity domain (right side)
    T1 = 0;              % A null generated thrust is assumed
    
elseif J0 < 0           % Out of linearity domain (left side)
    T1 = a1*abs(n1)*n1;    % Bollard thrust is assumed

else                    % Within the linearity domain
    T1 = a1*abs(n1)*n1 - a2*abs(n1)*V1;
end

== matlab function sim_all_2019b/Model/Vehicle Model/P2/Propeller2 ==
  data: n2 input; T2 output; V2 input; D parameter; omega parameter; a1 parameter; a2 parameter; alpha1 parameter; alpha2 parameter
function T2 = thrusterModel(n2, V2, D, omega, a1, a2, alpha1, alpha2)

Va2 = (1-omega) * V2;     % Advancement velocity at the propeller
J0 = Va2/(n2*D);          % Advancement Coefficient

if J0 > -alpha1/alpha2  % Out of linearity domain (right side)
    T2 = 0;              % A null generated thrust is assumed
    
elseif J0 < 0           % Out of linearity domain (left side)
    T2 = a1*abs(n2)*n2;    % Bollard thrust is assumed

else                    % Within the linearity domain
    T2 = a1*abs(n2)*n2 - a2*abs(n2)*V2;
end
